simulink model "Com_pedis"  (R2020b)
settings: Solver=VariableStepAuto  StartTime=0.0  StopTime=10.0  RelTol=1e-3
settings Model: Creator=Taha  LastModifiedBy=Taha

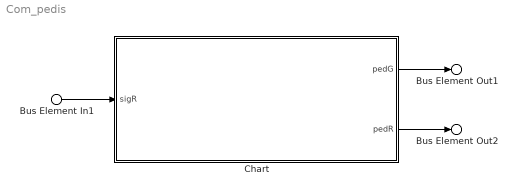
== system Com_pedis ==
  Bus Element In1 : Inport  PortName=sigR
  Chart : Stateflow chart  TreatAsAtomicUnit=on
  Bus Element Out1 : Outport  PortName=pedG
  Bus Element Out2 : Outport  Port=2  PortName=pedR
  wires:
  Bus Element In1/1 -> Chart/1(sigR)
  Chart/1(pedG) -> Bus Element Out1/1
  Chart/2(pedR) -> Bus Element Out2/1

== stateflow chart Com_pedis/Chart ==
  state GREEN
  state RED
  (default) -> GREEN : {pcount=0;}
  GREEN -> RED [order 1] : [pcount >= 55]{pedR = 1;}
  RED -> GREEN : [sigR == 1]{pedG = 1 ; pcount = 0;}
  GREEN -> GREEN [order 2] : {pcount = pcount + 1;}
  data: sigR input; pedG output; pedR output; pcount local
